simulink model "solenoid"  (Simulink 7.0)
settings: Solver=ode45  StartTime=0.0  StopTime=0.010  RelTol=1e-3
settings Model: Creator=binaryblade  LastModifiedBy=binaryblade

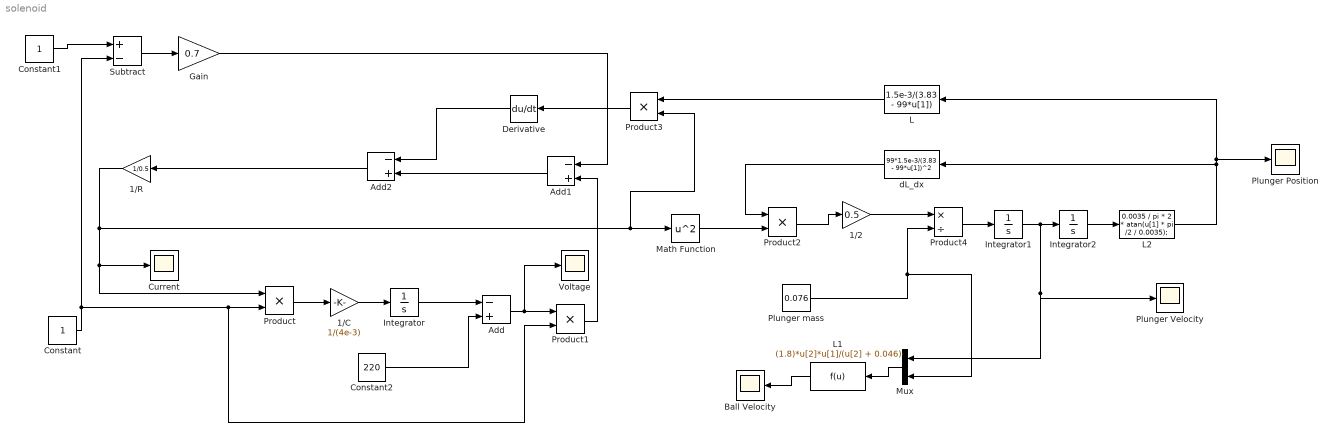
== system solenoid ==
  1/2 : Gain  Gain=0.5  ParameterDataType=sfix(16)  ParameterScaling=2^0  OutDataType=sfix(16)  OutScaling=2^0
  1/C : Gain  Gain=1/(4e-3)  ParameterDataType=sfix(16)  ParameterScaling=2^0  OutDataType=sfix(16)  OutScaling=2^0
  1/R : Gain  Orientation=left  Gain=1/0.5  ParameterDataType=sfix(16)  ParameterScaling=2^0  OutDataType=sfix(16)  OutScaling=2^0
  Add : Sum  Inputs=-+  OutDataType=sfix(16)  OutScaling=2^-10
  Add1 : Sum  Orientation=left  Inputs=-+  OutDataType=sfix(16)  OutScaling=2^-10
  Add2 : Sum  Orientation=left  Inputs=-+  OutDataType=sfix(16)  OutScaling=2^-10
  Ball Velocity : Scope
      settings: SaveName=ScopeData3
  Constant : Constant  OutDataType=sfix(16)  OutScaling=2^0
  Constant1 : Constant  OutDataType=sfix(16)  OutScaling=2^0
  Constant2 : Constant  Value=220  OutDataType=sfix(16)  OutScaling=2^0
  Current : Scope
  Derivative : Derivative  Orientation=left
  Gain : Gain  Gain=0.7  ParameterDataType=sfix(16)  ParameterScaling=2^0  OutDataType=sfix(16)  OutScaling=2^0
  Integrator : Integrator
  Integrator1 : Integrator
  Integrator2 : Integrator
  L : Fcn  Orientation=left  Expr=1.5e-3/(3.83 - 99*u[1])
  L1 : Fcn  Orientation=left  Expr=(1.8)*u[2]*u[1]/(u[2] + 0.046)
  L2 : Fcn  Expr=0.0035 / pi * 2 * atan(u[1] * pi /2 / 0.0035);
  Math Function : Math  Operator=square  OutDataType=sfix(16)  OutScaling=2^0  SaturateOnIntegerOverflow=on
  Mux : Mux  Orientation=left  Inputs=2
  Plunger Position : Scope
  Plunger Velocity : Scope
      settings: SaveName=ScopeData2
  Plunger mass : Constant  Value=0.076  OutDataType=sfix(16)  OutScaling=2^0
  Product : Product  OutDataType=sfix(16)  OutScaling=2^0  RndMeth=Zero
  Product1 : Product  OutDataType=sfix(16)  OutScaling=2^0  RndMeth=Zero
  Product2 : Product  OutDataType=sfix(16)  OutScaling=2^0  RndMeth=Zero
  Product3 : Product  Orientation=left  OutDataType=sfix(16)  OutScaling=2^0  RndMeth=Zero
  Product4 : Product  Inputs=*/  OutDataType=sfix(16)  OutScaling=2^0  RndMeth=Zero
  Subtract : Sum  Inputs=+-  OutDataType=sfix(16)  OutScaling=2^-10
  Voltage : Scope
      settings: SaveName=ScopeData4
  dL_dx : Fcn  Orientation=left  Expr=99*1.5e-3/(3.83 - 99*u[1])^2
  wires:
  Constant1/1 -> Subtract/1
  Constant/1 -> Subtract/2, Product/2, Product1/2
  Subtract/1 -> Gain/1
  Product/1 -> 1/C/1
  1/C/1 -> Integrator/1
  Integrator/1 -> Add/1
  Constant2/1 -> Add/2
  Add/1 -> Product1/1, Voltage/1
  Product1/1 -> Add1/2
  Gain/1 -> Add1/1
  Add1/1 -> Add2/2
  Add2/1 -> 1/R/1
  1/R/1 -> Product/1, Current/1, Math Function/1, Product3/2
  Derivative/1 -> Add2/1
  Math Function/1 -> Product2/2
  Product2/1 -> 1/2/1
  1/2/1 -> Product4/1
  Integrator1/1 -> Integrator2/1, Mux/1, Plunger Velocity/1
  Product3/1 -> Derivative/1
  L/1 -> Product3/1
  dL_dx/1 -> Product2/1
  Plunger mass/1 -> Product4/2, Mux/2
  L1/1 -> Ball Velocity/1
  Mux/1 -> L1/1
  Product4/1 -> Integrator1/1
  Integrator2/1 -> L2/1
  L2/1 -> Plunger Position/1, L/1, dL_dx/1
